simulink model "PolySim_IPRW_simulink"  (R2022b)
settings: Solver=VariableStepAuto  StartTime=0.0  StopTime=10  RelTol=1e-3
values from neighbouring files (symbols this model uses):
  A = [0, 1, 0; m_pend*g*L/Is, 0, Kt^2/(R*Is); 0, 0, -Kt^2/(R*Ir)]    [PolySim_IPRW_scriptV2.m]
  B = [0; -Kt/(R*Is); Kt/(R*Ir)]    [PolySim_IPRW_scriptV2.m]
  K_lqr = lqr(sys,Q,R_control)    [PolySim_IPRW_scriptV2.m]
  x0 = [deg2rad(i); 0; 0]    [PolySim_IPRW_scriptV2.m]
libraries: simulink x1
settings Model: Creator=natha  LastModifiedBy=ryanp

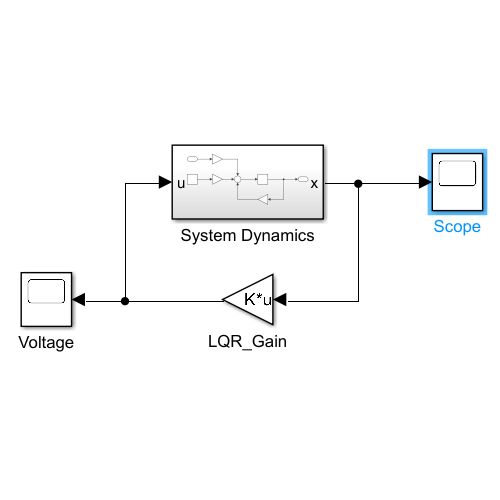
[thumbnail: Simulink's stored preview of the top-level diagram]
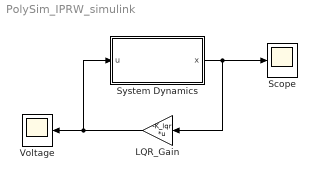
== system PolySim_IPRW_simulink ==
  LQR_Gain : Gain  Gain=-K_lqr  Multiplication=Matrix(K*u)
  Scope : Scope
  System Dynamics : Subsystem
  Voltage : Scope
  wires:
  LQR_Gain/1 -> Voltage/1, System Dynamics/1(u)
  System Dynamics/1(x) -> LQR_Gain/1, Scope/1

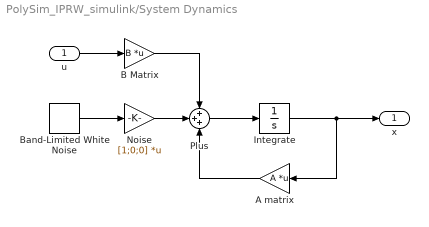
== system PolySim_IPRW_simulink/System Dynamics ==
  u : Inport
  A matrix : Gain  Gain=A  Multiplication=Matrix(K*u)
  B Matrix : Gain  Gain=B  Multiplication=Matrix(K*u)
  Band-Limited White Noise : simulink/Sources/Band-Limited White Noise  Cov=[0.1]  Ts=0.1  seed=[23341]
  Integrate : Integrator  InitialCondition=x0
  Noise : Gain  Gain=[1;0;0]  Multiplication=Matrix(K*u)
  Plus : Sum  Inputs=+++
  x : Outport
  wires:
  Plus/1 -> Integrate/1
  B Matrix/1 -> Plus/1
  Integrate/1 -> x/1, A matrix/1
  u/1 -> B Matrix/1
  A matrix/1 -> Plus/3
  Band-Limited White Noise/1 -> Noise/1
  Noise/1 -> Plus/2
